simulink model "main"  (R2020b)
settings: Solver=ode113  StartTime=0.0  StopTime=2*3600  RelTol=1e-13  AbsTol=1e-14
values from neighbouring files (symbols this model uses):
  Const = createSimulinkBus(Const_1)    [initializeData.m]
  Earth = createSimulinkBus(Earth_1)    [initializeData.m]
  Spacecraft = createSimulinkBus(Spacecraft_1)    [initializeData.m]
undefined symbols (not defined in the file or in its folder): initCond
libraries: SADlibrary x27, aerolibutil x7, sharedtransform x4, dspsrcs4 x3, sharedTrackingLibrary x3, vrlib x2, simulink_extras x2, sharedutil x1
(part 2 of 2)

== matlab function main/Real physics/Air drag/MATLAB Function ==
  data: F output; rho input; relVel input; T output; Spacecraft input
function [F,T] = getAirTorqueAndForce(rho, relVel, Spacecraft)

F = zeros(3,1);
T = zeros(3,1);

relVelMag = norm(relVel);
relVelDir = relVel/relVelMag;

for i = 1:size(Spacecraft.surfaces_normalToSurface,2)
    N_i = Spacecraft.surfaces_normalToSurface(:,i);
    A_i = Spacecraft.surfaces_area(:,i);
    r_i = Spacecraft.surfaces_position(:,i);
    Cd_i = Spacecraft.surfaces_Cd(i);
    
    F_i = dot(relVelDir,N_i);
    if F_i > 0
       F_i = F_i * 1/2*rho*Cd_i*relVelMag^2*A_i;
    else
       F_i = 0;
    end
    
    F = F - F_i * relVelDir;
    T = T - cross(r_i + Spacecraft.geometricCenter, F_i * relVelDir);
end

== matlab function main/Earth sensor reading/MATLAB Function ==
  data: theta input; A output; phi input; psi input
function A = rotationMatrix(theta,phi,psi)

A = [  cos(psi)*cos(theta)   cos(psi)*sin(theta)*sin(phi)+sin(psi)*cos(phi)  -cos(psi)*sin(theta)*cos(phi)+sin(psi)*sin(phi);
      -sin(psi)*cos(theta)  -sin(psi)*sin(theta)*sin(phi)+cos(psi)*cos(phi)   sin(psi)*sin(theta)*cos(phi)+cos(psi)*sin(phi);
                sin(theta)                             -cos(theta)*sin(phi)                              cos(theta)*cos(phi) ];

== matlab function main/Sun sensor reading/MATLAB Function ==
  data: theta input; A output; phi input; psi input
function A = rotationMatrix(theta,phi,psi)

A = [  cos(psi)*cos(theta)   cos(psi)*sin(theta)*sin(phi)+sin(psi)*cos(phi)  -cos(psi)*sin(theta)*cos(phi)+sin(psi)*sin(phi);
      -sin(psi)*cos(theta)  -sin(psi)*sin(theta)*sin(phi)+cos(psi)*cos(phi)   sin(psi)*sin(theta)*cos(phi)+cos(psi)*sin(phi);
                sin(theta)                             -cos(theta)*sin(phi)                              cos(theta)*cos(phi) ];

== matlab function main/MATLAB Function ==
  data: sunBF input size=3; A output size=[3 3]; sunECI input size=3; earthBF input size=3; earthECI input size=3
function A = getAttitude(sunBF,sunECI,earthBF,earthECI)

sunBF = sunBF / norm(sunBF);
sunECI = sunECI / norm(sunECI);

earthBF = earthBF / norm(earthBF);
earthECI = earthECI / norm(earthECI);

s1 = earthBF;
s2 = cross(earthBF,sunBF);
s2 = s2 / norm(s2);
s3 = cross(earthBF,s2);

v1 = earthECI;
v2 = cross(earthECI,sunECI);
v2 = v2 / norm(v2);
v3 = cross(earthECI,v2);

A = [s1 s2 s3]*[v1 v2 v3]';
% v = cross(sunBF,sunECI);
% theta = atan2(norm(v),dot(sunBF,sunECI));
% v = v / norm(v);
% q = [cos(theta/2);-sin(theta/2)*v];
% 
%

== matlab function main/MATLAB Function1 ==
  data: q input size=4; theta output size=1; v output size=3
function [theta,v] = fcn(q)

v = q(2:4);
vLen = norm(v);
v = v / vLen;
theta = atan2(q(1),vLen);
theta = theta*2;

== matlab function main/MATLAB Function2 ==
  data: sunBF input; A output; sunECI input; earthBF input; earthECI input
function A = getAttitude(sunBF,sunECI,earthBF,earthECI)

sunBF = sunBF / norm(sunBF);
sunECI = sunECI / norm(sunECI);

earthBF = earthBF / norm(earthBF);
earthECI = earthECI / norm(earthECI);

s1 = earthBF;
s2 = cross(earthBF,sunBF);
s2 = s2 / norm(s2);
s3 = cross(earthBF,s2);

v1 = earthECI;
v2 = cross(earthECI,sunECI);
v2 = v2 / norm(v2);
v3 = cross(earthECI,v2);

A = [s1 s2 s3]*[v1 v2 v3]';
% v = cross(sunBF,sunECI);
% theta = atan2(norm(v),dot(sunBF,sunECI));
% v = v / norm(v);
% q = [cos(theta/2);-sin(theta/2)*v];
% 
%

== matlab function main/MATLAB Function3 ==
  data: A_1_1 input; A output; A_1_2 input; A_1_3 input; A_2_1 input; A_2_2 input; A_2_3 input; A_3_1 input; A_3_2 input; A_3_3 input
function A = buildMatrix(A_1_1,A_1_2,A_1_3,A_2_1,A_2_2,A_2_3,A_3_1,A_3_2,A_3_3)

A = [A_1_1 A_1_2 A_1_3;...
     A_2_1 A_2_2 A_2_3;...
     A_3_1 A_3_2 A_3_3];
